simulink model "ControlDes"  (R2026a)
settings: Solver=ode3  StopTime=4  FixedStep=0.001  EnableMultiTasking=on
(part 1 of 12)
settings Model: Creator=fcbjo  LastModifiedBy=Mutti
settings SolverCC: ZeroCrossAlgorithm=Adaptive
settings DataIOCC: SaveState=on  InspectSignalLogs=on
settings OptimizationCC: StrengthReduction=on  OptimizationPriority=Speed  UseRestrictQualifier=on
settings DebuggingCC: MaskedZcDiagnostic=none  IgnoredZcDiagnostic=none  MultiTaskRateTransMsg=warning
settings HardwareCC: ProdLargestAtomicInteger=Long  ProdLargestAtomicFloat=Double  ProdHWDeviceType=ARM Compatible->ARM Cortex-M  TargetLargestAtomicInteger=Long  TargetLargestAtomicFloat=Double  TargetLongLongMode=on  TargetIntDivRoundTo=Zero  TargetEndianess=LittleEndian  TargetHWDeviceType=ARM Compatible->ARM Cortex-M
settings ModelReferenceCC: PropagateVarSize=During execution
settings RTWCC: SystemTargetFile=ert.tlc  GenCodeOnly=on  GenerateReport=on  BuildConfiguration=Faster Runs  IncludeHyperlinkInReport=on  LaunchReport=on  PortableWordSizes=on  CodeProfilingSaveOptions=AllData  TargetLang=C++  GenerateTraceInfo=on  GenerateTraceReport=on  GenerateTraceReportSl=on  GenerateTraceReportSf=on  GenerateTraceReportEml=on  GenerateWebview=on  GenerateCodeMetricsReport=on  GenerateCodeReplacementReport=on  Description=Embedded Coder
settings CodeAppCC: GenerateComments=off
settings ERTTargetCC: RootIOFormat=Structure reference  TargetLangStandard=C++20 (ISO)  CodeReplacementLibrary=ARM Cortex-M  CodeInterfacePackaging=C++ class  SubcomponentCodeInterfacePackaging=C++ class  SupportNonFinite=off  SupportVariableSizeSignals=on

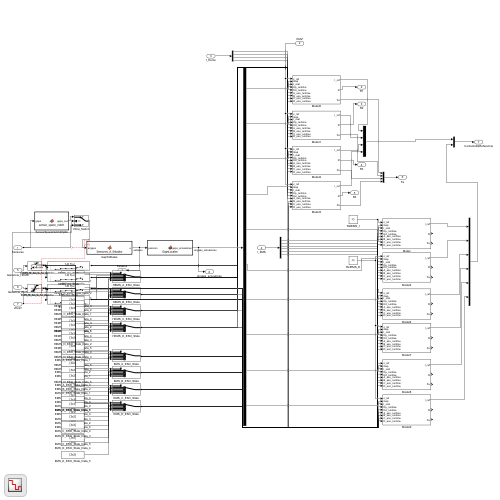
[thumbnail: Simulink's stored preview of the top-level diagram]
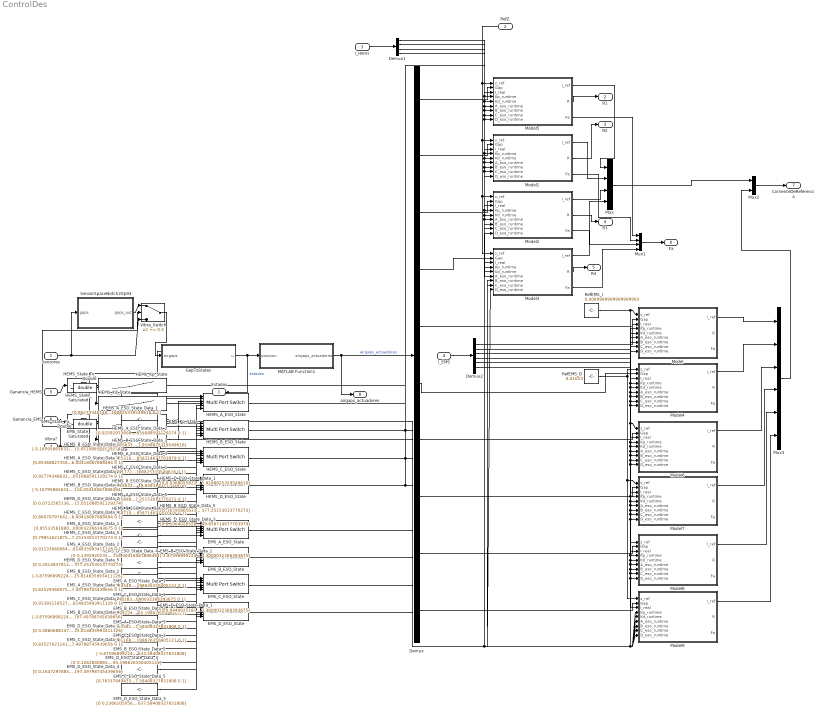
== system ControlDes ==
  Sensores : Inport  OutDataTypeStr=double  PortDimensions=8  SampleTime=[0.001,0]
  RefZ : Inport  Port=2  OutDataTypeStr=double  PortDimensions=1
  I_Hems : Inport  Port=3  OutDataTypeStr=double  PortDimensions=4  SampleTime=[0.001,0]
  I_EMS : Inport  Port=4
  Ganancia_HEMS : Inport  Port=5  OutDataTypeStr=uint8
  Ganancia_EMS : Inport  Port=6  OutDataTypeStr=uint8
  Vibra? : Inport  Port=7  OutDataTypeStr=boolean
  Demux : Demux  Outputs=10
  Demux1 : Demux
  Demux2 : Demux  Outputs=6
  EMS_A_ESO_State : MultiPortSwitch  Inputs=5  SaturateOnIntegerOverflow=off  InputSameDT=off
  EMS_A_ESO_State_Data_1 : Constant  Value=[0.95533581880918794 0.001 4.9999999999999998e-07;-0.66331302553024352 1 0.001;-3.3000032366393675 0 1]
  EMS_A_ESO_State_Data_2 : Constant  Value=[0.91133660064552446 0.001 4.9999999999999998e-07;-2.6074920437003652 1 0.001;-25.814835993411126 0 1]
  EMS_A_ESO_State_Data_3 : Constant  Value=[0.86799244549929988 0.001 4.9999999999999998e-07;-5.7660655019099014 1 0.001;-85.198626350405121 0 1]
  EMS_A_ESO_State_Data_4 : Constant  Value=[0.82529360075274616 0.001 4.9999999999999998e-07;-10.075359652253088 1 0.001;-197.49798745439656 0 1]
  EMS_A_ESO_State_Data_5 : Constant  Value=[0.74179355581368456 0.001 4.9999999999999998e-07;-21.904730564807785 1 0.001;-637.58408327831808 0 1]
  EMS_B_ESO_State : MultiPortSwitch  Inputs=5  SaturateOnIntegerOverflow=off  InputSameDT=off
  EMS_B_ESO_State_Data_1 : Constant  Value=[-3.8759689922480615e-09 0.044664181190812058;-7.7519379844961241e-06 0.66331302553024352;0 3.3000032366393675]
  EMS_B_ESO_State_Data_2 : Constant  Value=[-3.8759689922480615e-09 0.088663399354475536;-7.7519379844961241e-06 2.6074920437003652;0 25.814835993411126]
  EMS_B_ESO_State_Data_3 : Constant  Value=[-3.8759689922480615e-09 0.13200755450070012;-7.7519379844961241e-06 5.7660655019099014;0 85.198626350405121]
  EMS_B_ESO_State_Data_4 : Constant  Value=[-3.8759689922480615e-09 0.17470639924725384;-7.7519379844961241e-06 10.075359652253088;0 197.49798745439656]
  EMS_B_ESO_State_Data_5 : Constant  Value=[-3.8759689922480615e-09 0.25820644418631544;-7.7519379844961241e-06 21.904730564807785;0 637.58408327831808]
  EMS_C_ESO_State : MultiPortSwitch  Inputs=5  SaturateOnIntegerOverflow=off  InputSameDT=off
  EMS_C_ESO_State_Data_1 : Constant  Value=[0.95599748183309985 0 0;-0.66001302229360415 1 0;-3.3000032366393675 0 1]
  EMS_C_ESO_State_Data_2 : Constant  Value=[0.91393118527122807 0 0;-2.5816772077069543 1 0;-25.814835993411126 0 1]
  EMS_C_ESO_State_Data_3 : Constant  Value=[0.87371591168803464 0 0;-5.680866875559496 1 0;-85.198626350405121 0 1]
  EMS_C_ESO_State_Data_4 : Constant  Value=[0.835270211411272 0 0;-9.8778616647986919 1 0;-197.49798745439656 0 1]
  EMS_C_ESO_State_Data_5 : Constant  Value=[0.76337949433685315 0 0;-21.267146481529466 1 0;-637.58408327831808 0 1]
  EMS_D_ESO_State : MultiPortSwitch  Inputs=5  SaturateOnIntegerOverflow=off  InputSameDT=off
  EMS_D_ESO_State_Data_1 : Constant  Value=[0 0.04400251816690013;0 0.66001302229360415;0 3.3000032366393675]
  EMS_D_ESO_State_Data_2 : Constant  Value=[0 0.086068814728771884;0 2.5816772077069543;0 25.814835993411126]
  EMS_D_ESO_State_Data_3 : Constant  Value=[0 0.12628408831196541;0 5.680866875559496;0 85.198626350405121]
  EMS_D_ESO_State_Data_4 : Constant  Value=[0 0.16472978858872794;0 9.8778616647986919;0 197.49798745439656]
  EMS_D_ESO_State_Data_5 : Constant  Value=[0 0.23662050566314682;0 21.267146481529466;0 637.58408327831808]
  EMS_Kd_State : Lookup_n-D  NumberOfTableDimensions=1  BreakpointsForDimension1=[1 2 3 4 5]  IndexSearchMethod=Evenly spaced points  Table=[10 20 30 40 60]  InterpMethod=Flat  ExtrapMethod=Clip  InternalRulePriority=Speed  RndMeth=Simplest
  EMS_Kp_State : Lookup_n-D  NumberOfTableDimensions=1  BreakpointsForDimension1=[1 2 3 4 5]  IndexSearchMethod=Evenly spaced points  Table=[25 100 225 400 900]  InterpMethod=Flat  ExtrapMethod=Clip  InternalRulePriority=Speed  RndMeth=Simplest
  EMS_State_Saturated : Saturate  UpperLimit=5  LowerLimit=1
  EMS_State_To_Double : DataTypeConversion  OutDataTypeStr=double  SaturateOnIntegerOverflow=off  RndMeth=Floor
  GapToStates : MATLAB Function  TreatAsAtomicUnit=on
  HEMS_A_ESO_State : MultiPortSwitch  Inputs=5  SaturateOnIntegerOverflow=off  InputSameDT=off
  HEMS_A_ESO_State_Data_1 : Constant  Value=[0.96273340148164432 0.001 4.9999999999999998e-07;-0.46197468044345896 1 0.001;-1.9168825319549616 0 1]
  HEMS_A_ESO_State_Data_2 : Constant  Value=[0.92592973608499785 0.001 4.9999999999999998e-07;-1.8212757878504588 1 0.001;-15.051088591129274 0 1]
  HEMS_A_ESO_State_Data_3 : Constant  Value=[0.88958325316246545 0.001 4.9999999999999998e-07;-4.0390233033892127 1 0.001;-49.858714677703979 0 1]
  HEMS_A_ESO_State_Data_4 : Constant  Value=[0.85368827350214205 0.001 4.9999999999999998e-07;-7.0777050132552208 1 0.001;-116.00418067888494 0 1]
  HEMS_A_ESO_State_Data_5 : Constant  Value=[0.78323045898565857 0.001 4.9999999999999998e-07;-15.474385538787232 1 0.001;-377.25153013770273 0 1]
  HEMS_B_ESO_State : MultiPortSwitch  Inputs=5  SaturateOnIntegerOverflow=off  InputSameDT=off
  HEMS_B_ESO_State_Data_1 : Constant  Value=[-5.1679586563307495e-09 0.037266598518355676;-1.0335917312661499e-05 0.46197468044345896;0 1.9168825319549616]
  HEMS_B_ESO_State_Data_2 : Constant  Value=[-5.1679586563307495e-09 0.074070263915002155;-1.0335917312661499e-05 1.8212757878504588;0 15.051088591129274]
  HEMS_B_ESO_State_Data_3 : Constant  Value=[-5.1679586563307495e-09 0.11041674683753455;-1.0335917312661499e-05 4.0390233033892127;0 49.858714677703979]
  HEMS_B_ESO_State_Data_4 : Constant  Value=[-5.1679586563307495e-09 0.14631172649785795;-1.0335917312661499e-05 7.0777050132552208;0 116.00418067888494]
  HEMS_B_ESO_State_Data_5 : Constant  Value=[-5.1679586563307495e-09 0.21676954101434143;-1.0335917312661499e-05 15.474385538787232;0 377.25153013770273]
  HEMS_C_ESO_State : MultiPortSwitch  Inputs=5  SaturateOnIntegerOverflow=off  InputSameDT=off
  HEMS_C_ESO_State_Data_1 : Constant  Value=[0.96319441772082182 0 0;-0.46005779791150397 1 0;-1.9168825319549616 0 1]
  HEMS_C_ESO_State_Data_2 : Constant  Value=[0.92774348632855275 0 0;-1.8062246992593296 1 0;-15.051088591129274 0 1]
  HEMS_C_ESO_State_Data_3 : Constant  Value=[0.89359734710851579 0 0;-3.9891645887115086 1 0;-49.858714677703979 0 1]
  HEMS_C_ESO_State_Data_4 : Constant  Value=[0.86070797642505781 0 0;-6.9617008325763363 1 0;-116.00418067888494 0 1]
  HEMS_C_ESO_State_Data_5 : Constant  Value=[0.79851621875937695 0 0;-15.09713400864953 1 0;-377.25153013770273 0 1]
  HEMS_D_ESO_State : MultiPortSwitch  Inputs=5  SaturateOnIntegerOverflow=off  InputSameDT=off
  HEMS_D_ESO_State_Data_1 : Constant  Value=[0 0.036805582279178198;0 0.46005779791150397;0 1.9168825319549616]
  HEMS_D_ESO_State_Data_2 : Constant  Value=[0 0.072256513671447267;0 1.8062246992593296;0 15.051088591129274]
  HEMS_D_ESO_State_Data_3 : Constant  Value=[0 0.10640265289148419;0 3.9891645887115086;0 49.858714677703979]
  HEMS_D_ESO_State_Data_4 : Constant  Value=[0 0.13929202357494219;0 6.9617008325763363;0 116.00418067888494]
  HEMS_D_ESO_State_Data_5 : Constant  Value=[0 0.20148378124062305;0 15.09713400864953;0 377.25153013770273]
  HEMS_Kd_State : Lookup_n-D  NumberOfTableDimensions=1  BreakpointsForDimension1=[1 2 3 4 5]  IndexSearchMethod=Evenly spaced points  Table=[10 20 30 40 60]  InterpMethod=Flat  ExtrapMethod=Clip  InternalRulePriority=Speed  RndMeth=Simplest
  HEMS_Kp_State : Lookup_n-D  NumberOfTableDimensions=1  BreakpointsForDimension1=[1 2 3 4 5]  IndexSearchMethod=Evenly spaced points  Table=[25 100 225 400 900]  InterpMethod=Flat  ExtrapMethod=Clip  InternalRulePriority=Speed  RndMeth=Simplest
  HEMS_State_Saturated : Saturate  UpperLimit=5  LowerLimit=1
  HEMS_State_To_Double : DataTypeConversion  OutDataTypeStr=double  SaturateOnIntegerOverflow=off  RndMeth=Floor
  MATLAB Function1 : MATLAB Function  TreatAsAtomicUnit=on
  Model : Subsystem
  Model1 : Subsystem
  Model2 : Subsystem
  Model3 : Subsystem
  Model4 : Subsystem
  Model5 : Subsystem
  Model6 : Subsystem
  Model7 : Subsystem
  Model8 : Subsystem
  Model9 : Subsystem
  Mux : Mux
  Mux1 : Mux
  Mux2 : Mux  Inputs=2
  Mux3 : Mux  Inputs=6
  RefEMS_D : Constant  Value=0.01023
  RefEMS_I : Constant  Value=0.0089999999999999993
  SensorSpaceNotch20p94 : MATLAB Function  TreatAsAtomicUnit=on
  Vibra_Switch : Switch  Threshold=0.5  SaturateOnIntegerOverflow=off  InputSameDT=off
  Estados : Outport  OutDataTypeStr=double  PortDimensions=[5 1]  SampleTime=[0.001,0]
  R1 : Outport  Port=2  OutDataTypeStr=double  PortDimensions=3  SampleTime=[0.001,0]
  R2 : Outport  Port=3  OutDataTypeStr=double  PortDimensions=3  SampleTime=[0.001,0]
  R3 : Outport  Port=4  OutDataTypeStr=double  PortDimensions=3  SampleTime=[0.001,0]
  R4 : Outport  Port=5  OutDataTypeStr=double  PortDimensions=3  SampleTime=[0.001,0]
  Fa : Outport  Port=6  OutDataTypeStr=double  PortDimensions=4  SampleTime=[0.001,0]
  CorrienteDeReferencia : Outport  Port=7
  airgaps_actuadores : Outport  Port=8
  wires:
  GapToStates/1(u) -> MATLAB Function1/1(posicion), Estados/1  "estados"
  MATLAB Function1/1(airgaps_actuadores) -> airgaps_actuadores/1, Demux/1  "airgaps_actuadores"
  RefZ/1 -> Model2/1(z_ref), Model3/1(z_ref), Model1/1(z_ref), Model5/1(z_ref)
  I_Hems/1 -> Demux1/1
  Mux1/1 -> Fa/1
  RefEMS_I/1 -> Model6/1(z_ref), Model8/1(z_ref), Model/1(z_ref)
  I_EMS/1 -> Demux2/1
  Mux2/1 -> CorrienteDeReferencia/1
  Mux/1 -> Mux2/1
  Mux3/1 -> Mux2/2
  RefEMS_D/1 -> Model7/1(z_ref), Model9/1(z_ref), Model4/1(z_ref)
  Demux/5 -> Model/2(Gap)
  Demux2/1 -> Model/3(I_real)
  Model/1(I_ref) -> Mux3/1
  Demux/2 -> Model1/2(Gap)
  Demux1/2 -> Model1/3(I_real)
  Model1/1(I_ref) -> Mux/2
  Model1/2(R) -> R2/1
  Model1/3(Fa) -> Mux1/2
  Demux/3 -> Model2/2(Gap)
  Demux1/3 -> Model2/3(I_real)
  Model2/1(I_ref) -> Mux/3
  Model2/2(R) -> R3/1
  Model2/3(Fa) -> Mux1/3
  Demux/4 -> Model3/2(Gap)
  Demux1/4 -> Model3/3(I_real)
  Model3/1(I_ref) -> Mux/4
  Model3/2(R) -> R4/1
  Model3/3(Fa) -> Mux1/4
  Demux/6 -> Model4/2(Gap)
  Demux2/2 -> Model4/3(I_real)
  Model4/1(I_ref) -> Mux3/2
  Demux/1 -> Model5/2(Gap)
  Demux1/1 -> Model5/3(I_real)
  Model5/1(I_ref) -> Mux/1
  Model5/2(R) -> R1/1
  Model5/3(Fa) -> Mux1/1
  Demux/7 -> Model6/2(Gap)
  Demux2/3 -> Model6/3(I_real)
  Model6/1(I_ref) -> Mux3/3
  Demux/8 -> Model7/2(Gap)
  Demux2/4 -> Model7/3(I_real)
  Model7/1(I_ref) -> Mux3/4
  Demux/9 -> Model8/2(Gap)
  Demux2/5 -> Model8/3(I_real)
  Model8/1(I_ref) -> Mux3/5
  Demux/10 -> Model9/2(Gap)
  Demux2/6 -> Model9/3(I_real)
  Model9/1(I_ref) -> Mux3/6
  HEMS_Kp_State/1 -> Model2/4(Kp_runtime), Model3/4(Kp_runtime), Model1/4(Kp_runtime), Model5/4(Kp_runtime)
  HEMS_Kd_State/1 -> Model2/5(Kd_runtime), Model3/5(Kd_runtime), Model1/5(Kd_runtime), Model5/5(Kd_runtime)
  EMS_Kp_State/1 -> Model/4(Kp_runtime), Model4/4(Kp_runtime), Model6/4(Kp_runtime), Model7/4(Kp_runtime), Model8/4(Kp_runtime), Model9/4(Kp_runtime)
  EMS_Kd_State/1 -> Model/5(Kd_runtime), Model4/5(Kd_runtime), Model6/5(Kd_runtime), Model7/5(Kd_runtime), Model8/5(Kd_runtime), Model9/5(Kd_runtime)
  ? -> ?
  Vibra?/1 -> Vibra_Switch/2
  Ganancia_HEMS/1 -> HEMS_State_Saturated/1
  HEMS_State_To_Double/1 -> HEMS_Kp_State/1, HEMS_Kd_State/1
  Ganancia_EMS/1 -> EMS_State_Saturated/1
  EMS_State_To_Double/1 -> EMS_Kp_State/1, EMS_Kd_State/1
  HEMS_State_Saturated/1 -> HEMS_C_ESO_State/1, HEMS_D_ESO_State/1, HEMS_B_ESO_State/1, HEMS_A_ESO_State/1, HEMS_State_To_Double/1
  EMS_State_Saturated/1 -> EMS_C_ESO_State/1, EMS_D_ESO_State/1, EMS_B_ESO_State/1, EMS_A_ESO_State/1, EMS_State_To_Double/1
  HEMS_A_ESO_State_Data_1/1 -> HEMS_A_ESO_State/2
  HEMS_A_ESO_State_Data_2/1 -> HEMS_A_ESO_State/3
  HEMS_A_ESO_State_Data_3/1 -> HEMS_A_ESO_State/4
  HEMS_A_ESO_State_Data_4/1 -> HEMS_A_ESO_State/5
  HEMS_A_ESO_State_Data_5/1 -> HEMS_A_ESO_State/6
  HEMS_B_ESO_State_Data_1/1 -> HEMS_B_ESO_State/2
  HEMS_B_ESO_State_Data_2/1 -> HEMS_B_ESO_State/3
  HEMS_B_ESO_State_Data_3/1 -> HEMS_B_ESO_State/4
  HEMS_B_ESO_State_Data_4/1 -> HEMS_B_ESO_State/5
  HEMS_B_ESO_State_Data_5/1 -> HEMS_B_ESO_State/6
  HEMS_C_ESO_State_Data_1/1 -> HEMS_C_ESO_State/2
  HEMS_C_ESO_State_Data_2/1 -> HEMS_C_ESO_State/3
  HEMS_C_ESO_State_Data_3/1 -> HEMS_C_ESO_State/4
  HEMS_C_ESO_State_Data_4/1 -> HEMS_C_ESO_State/5
  HEMS_C_ESO_State_Data_5/1 -> HEMS_C_ESO_State/6
  HEMS_D_ESO_State_Data_1/1 -> HEMS_D_ESO_State/2
  HEMS_D_ESO_State_Data_2/1 -> HEMS_D_ESO_State/3
  HEMS_D_ESO_State_Data_3/1 -> HEMS_D_ESO_State/4
  HEMS_D_ESO_State_Data_4/1 -> HEMS_D_ESO_State/5
  HEMS_D_ESO_State_Data_5/1 -> HEMS_D_ESO_State/6
  EMS_A_ESO_State_Data_1/1 -> EMS_A_ESO_State/2
  EMS_A_ESO_State_Data_2/1 -> EMS_A_ESO_State/3
  EMS_A_ESO_State_Data_3/1 -> EMS_A_ESO_State/4
  EMS_A_ESO_State_Data_4/1 -> EMS_A_ESO_State/5
  EMS_A_ESO_State_Data_5/1 -> EMS_A_ESO_State/6
  EMS_B_ESO_State_Data_1/1 -> EMS_B_ESO_State/2
  EMS_B_ESO_State_Data_2/1 -> EMS_B_ESO_State/3
  EMS_B_ESO_State_Data_3/1 -> EMS_B_ESO_State/4
  EMS_B_ESO_State_Data_4/1 -> EMS_B_ESO_State/5
  EMS_B_ESO_State_Data_5/1 -> EMS_B_ESO_State/6
  EMS_C_ESO_State_Data_1/1 -> EMS_C_ESO_State/2
  EMS_C_ESO_State_Data_2/1 -> EMS_C_ESO_State/3
  EMS_C_ESO_State_Data_3/1 -> EMS_C_ESO_State/4
  EMS_C_ESO_State_Data_4/1 -> EMS_C_ESO_State/5
  EMS_C_ESO_State_Data_5/1 -> EMS_C_ESO_State/6
  EMS_D_ESO_State_Data_1/1 -> EMS_D_ESO_State/2
  EMS_D_ESO_State_Data_2/1 -> EMS_D_ESO_State/3
  EMS_D_ESO_State_Data_3/1 -> EMS_D_ESO_State/4
  EMS_D_ESO_State_Data_4/1 -> EMS_D_ESO_State/5
  EMS_D_ESO_State_Data_5/1 -> EMS_D_ESO_State/6
  HEMS_A_ESO_State/1 -> Model2/6(A_eso_runtime), Model3/6(A_eso_runtime), Model1/6(A_eso_runtime), Model5/6(A_eso_runtime)
  HEMS_B_ESO_State/1 -> Model1/7(B_eso_runtime), Model2/7(B_eso_runtime), Model5/7(B_eso_runtime), Model3/7(B_eso_runtime)
  HEMS_C_ESO_State/1 -> Model1/8(C_eso_runtime), Model2/8(C_eso_runtime), Model5/8(C_eso_runtime), Model3/8(C_eso_runtime)
  HEMS_D_ESO_State/1 -> Model2/9(D_eso_runtime), Model3/9(D_eso_runtime), Model1/9(D_eso_runtime), Model5/9(D_eso_runtime)
  EMS_A_ESO_State/1 -> Model/6(A_eso_runtime), Model4/6(A_eso_runtime), Model6/6(A_eso_runtime), Model7/6(A_eso_runtime), Model8/6(A_eso_runtime), Model9/6(A_eso_runtime)
  EMS_B_ESO_State/1 -> Model/7(B_eso_runtime), Model4/7(B_eso_runtime), Model6/7(B_eso_runtime), Model7/7(B_eso_runtime), Model8/7(B_eso_runtime), Model9/7(B_eso_runtime)
  EMS_C_ESO_State/1 -> Model/8(C_eso_runtime), Model4/8(C_eso_runtime), Model6/8(C_eso_runtime), Model7/8(C_eso_runtime), Model8/8(C_eso_runtime), Model9/8(C_eso_runtime)
  EMS_D_ESO_State/1 -> Model/9(D_eso_runtime), Model4/9(D_eso_runtime), Model6/9(D_eso_runtime), Model7/9(D_eso_runtime), Model8/9(D_eso_runtime), Model9/9(D_eso_runtime)
  Sensores/1 -> SensorSpaceNotch20p94/1(gaps), Vibra_Switch/3
  SensorSpaceNotch20p94/1(gaps_out) -> Vibra_Switch/1
  Vibra_Switch/1 -> GapToStates/1(airgaps)
